simulink subsystem "MotoresJGV"  (R2024b)
settings: Solver=VariableStepAuto  StartTime=0.0  StopTime=10.0  RelTol=1e-3
libraries: arduinolib x6
settings Model: Creator=USUARIO  LastModifiedBy=USUARIO

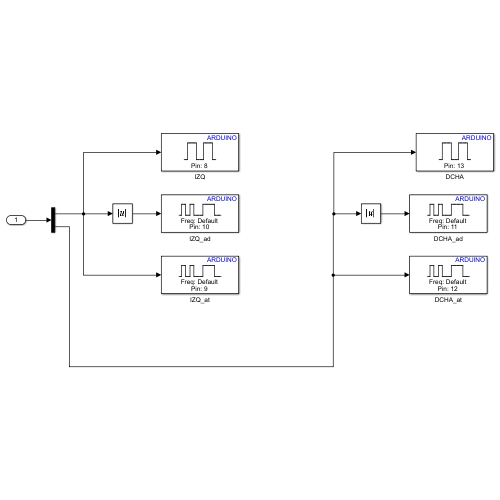
[thumbnail: Simulink's stored preview of the top-level diagram]
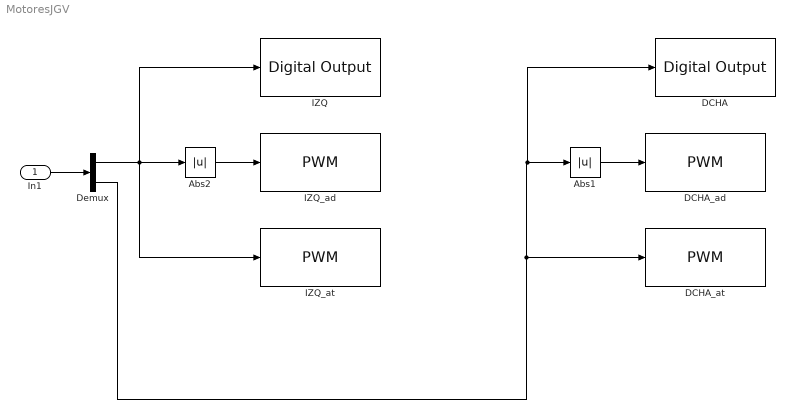
== system MotoresJGV ==
  In1 : Inport
  Abs1 : Abs  SaturateOnIntegerOverflow=off
  Abs2 : Abs  SaturateOnIntegerOverflow=off
  DCHA : arduinolib/Digital Output  pinNumber=13  Direction=output  blockPlatform=arduino
  DCHA_ad : arduinolib/PWM  pinNumber=11  frequencyType=Default  desiredFrequency=490.2  achievableFrequency=490.2
  DCHA_at : arduinolib/PWM  pinNumber=12  frequencyType=Default  desiredFrequency=490.2  achievableFrequency=490.2
  Demux : Demux  Outputs=2
  IZQ : arduinolib/Digital Output  pinNumber=8  Direction=output  blockPlatform=arduino
  IZQ_ad : arduinolib/PWM  pinNumber=10  frequencyType=Default  desiredFrequency=490.2  achievableFrequency=490.2
  IZQ_at : arduinolib/PWM  pinNumber=9  frequencyType=Default  desiredFrequency=490.2  achievableFrequency=490.2
  wires:
  Demux/1 -> IZQ_at/1, IZQ/1, Abs2/1
  Demux/2 -> DCHA_at/1, DCHA/1, Abs1/1
  In1/1 -> Demux/1
  Abs1/1 -> DCHA_ad/1
  Abs2/1 -> IZQ_ad/1
